simulink model "comm_test"  (R2021a)
settings: Solver=FixedStepAuto  StartTime=0.0  StopTime=inf  RelTol=1e-3
model workspace (MAT data in the model file):
  SL_ROS_VariableLengthArrays_MaxSizes.CommonInfo.ArrayTruncateAction = 'EmitWarning'
  SL_ROS_VariableLengthArrays_MaxSizes.MsgTypeMap = containers.Map
  SL_ROS_VariableLengthArrays_MaxSizes.MsgTypeMap.serialization.keys = {'ambf_walker/DesiredJoints', 'sensor_msgs/JointState'}
  SL_ROS_VariableLengthArrays_MaxSizes.MsgTypeMap.serialization.values{1}(1).PropertyName = 'Controller'
  SL_ROS_VariableLengthArrays_MaxSizes.MsgTypeMap.serialization.values{1}(1).DataType = 'uint8'
  SL_ROS_VariableLengthArrays_MaxSizes.MsgTypeMap.serialization.values{1}(1).MaxLength = 128
  SL_ROS_VariableLengthArrays_MaxSizes.MsgTypeMap.serialization.values{1}(2).PropertyName = 'Other'
  SL_ROS_VariableLengthArrays_MaxSizes.MsgTypeMap.serialization.values{1}(2).DataType = 'double'
  SL_ROS_VariableLengthArrays_MaxSizes.MsgTypeMap.serialization.values{1}(2).MaxLength = 7
  SL_ROS_VariableLengthArrays_MaxSizes.MsgTypeMap.serialization.values{1}(3).PropertyName = 'Q'
  SL_ROS_VariableLengthArrays_MaxSizes.MsgTypeMap.serialization.values{1}(3).DataType = 'double'
  SL_ROS_VariableLengthArrays_MaxSizes.MsgTypeMap.serialization.values{1}(3).MaxLength = 7
  SL_ROS_VariableLengthArrays_MaxSizes.MsgTypeMap.serialization.values{1}(4).PropertyName = 'Qd'
  SL_ROS_VariableLengthArrays_MaxSizes.MsgTypeMap.serialization.values{1}(4).DataType = 'double'
  SL_ROS_VariableLengthArrays_MaxSizes.MsgTypeMap.serialization.values{1}(4).MaxLength = 7
  SL_ROS_VariableLengthArrays_MaxSizes.MsgTypeMap.serialization.values{1}(5).PropertyName = 'Qdd'
  SL_ROS_VariableLengthArrays_MaxSizes.MsgTypeMap.serialization.values{1}(5).DataType = 'double'
  SL_ROS_VariableLengthArrays_MaxSizes.MsgTypeMap.serialization.values{1}(5).MaxLength = 7
  SL_ROS_VariableLengthArrays_MaxSizes.MsgTypeMap.serialization.values{2}(1).PropertyName = 'Effort'
  SL_ROS_VariableLengthArrays_MaxSizes.MsgTypeMap.serialization.values{2}(1).DataType = 'double'
  SL_ROS_VariableLengthArrays_MaxSizes.MsgTypeMap.serialization.values{2}(1).MaxLength = 7
  SL_ROS_VariableLengthArrays_MaxSizes.MsgTypeMap.serialization.values{2}(2).PropertyName = 'Name'
  SL_ROS_VariableLengthArrays_MaxSizes.MsgTypeMap.serialization.values{2}(2).DataType = 'std_msgs/String'
  SL_ROS_VariableLengthArrays_MaxSizes.MsgTypeMap.serialization.values{2}(2).MaxLength = 7
  SL_ROS_VariableLengthArrays_MaxSizes.MsgTypeMap.serialization.values{2}(3).PropertyName = 'Position'
  SL_ROS_VariableLengthArrays_MaxSizes.MsgTypeMap.serialization.values{2}(3).DataType = 'double'
  SL_ROS_VariableLengthArrays_MaxSizes.MsgTypeMap.serialization.values{2}(3).MaxLength = 7
  SL_ROS_VariableLengthArrays_MaxSizes.MsgTypeMap.serialization.values{2}(4).PropertyName = 'Velocity'
  SL_ROS_VariableLengthArrays_MaxSizes.MsgTypeMap.serialization.values{2}(4).DataType = 'double'
  SL_ROS_VariableLengthArrays_MaxSizes.MsgTypeMap.serialization.values{2}(4).MaxLength = 7
  SL_ROS_VariableLengthArrays_MaxSizes.MsgTypeMap.serialization.uniformity = 0
  SL_ROS_VariableLengthArrays_MaxSizes.MsgTypeMap.serialization.keyType = 'char'
  SL_ROS_VariableLengthArrays_MaxSizes.MsgTypeMap.serialization.valueType = 'any'
values from neighbouring files (symbols this model uses):
  Kd = eye(7)*10    [PD_controller_setup.m]    (also in sliding_controller_init.m = 50*eye(7))
  Kp = eye(7)*10    [PD_controller_setup.m]
libraries: robotlib x12
settings Model: Creator=nathanielgoldfarb  LastModifiedBy=nathanielgoldfarb
settings OptimizationCC: EnhancedBackFolding=on  PassReuseOutputArgsAs=Individual arguments  ZeroExternalMemoryAtStartup=off  ZeroInternalMemoryAtStartup=off  MaxStackSize=64  OptimizeBlockOrder=speed  DifferentSizesBufferReuse=on  OptimizationCustomize=off  EfficientTunableParamExpr=on
settings DebuggingCC: ParameterTunabilityLossMsg=error
settings HardwareCC: ProdBitPerPointer=32  ProdBitPerSizeT=32  ProdBitPerPtrDiffT=32  ProdLargestAtomicFloat=None  ProdIntDivRoundTo=Undefined  ProdEndianess=Unspecified  ProdWordSize=32  ProdHWDeviceType=Generic->Unspecified (assume 32-bit Generic)  UseEmbeddedCoderFeatures=off
settings SFSimCC: MATLABDynamicMemAlloc=off
settings RTWCC: SystemTargetFile=ert.tlc  HardwareBoard=Robot Operating System (ROS)  TLCOptions="-aInlineSetEventsForThisBaseRateFcn=TLC_FALSE -aSuppressMultiTaskScheduler=TLC_FALSE  -aRateBasedStepFcn=0"  TemplateMakefile=ert_default_tmf  Toolchain=Catkin  TargetLang=C++
settings CodeAppCC: ForceParamTrailComments=on  IgnoreCustomStorageClasses=off  OperatorAnnotations=on  SimulinkDataObjDesc=on  SFDataObjDesc=on  InsertBlockDesc=on
settings ERTTargetCC: SupportNonInlinedSFcns=on

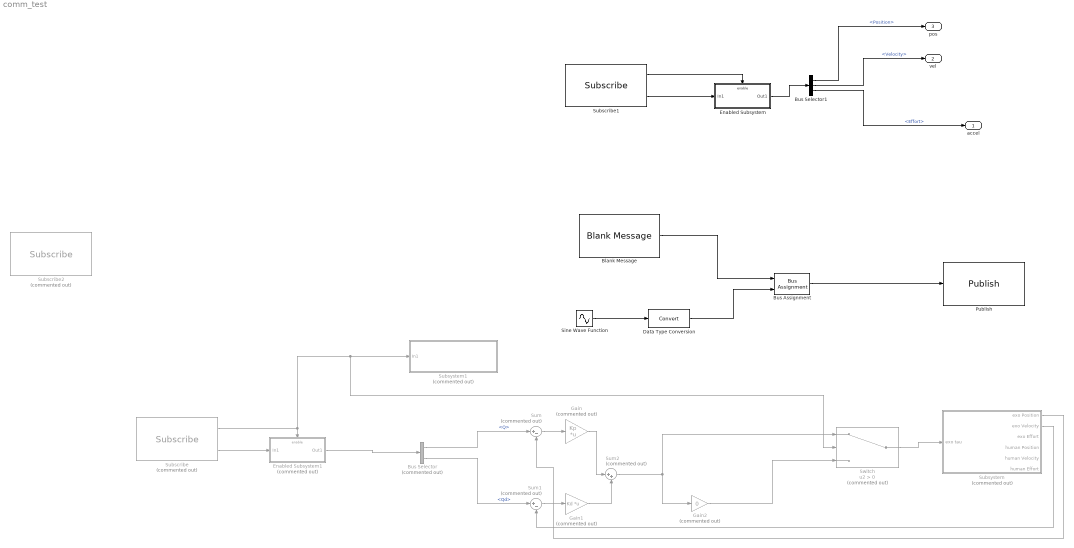
== system comm_test ==
  Blank Message : robotlib/Blank Message  messageClass=Message  entityType=std_msgs/Float32  messageType=std_msgs/Float32  SampleTime=-1  legacyBusStruct=off
  Bus Assignment : BusAssignment  AssignedSignals=Data
  Bus Selector : BusSelector  Commented=on  OutputSignals=Q,Qd
  Bus Selector1 : BusSelector  OutputSignals=Position,Velocity,Effort
  Data Type Conversion : DataTypeConversion
  Enabled Subsystem : Subsystem  TreatAsAtomicUnit=on
  Enabled Subsystem1 : Subsystem  Commented=on  TreatAsAtomicUnit=on
  Gain : Gain  Commented=on  Gain=Kp  Multiplication=Matrix(K*u)
  Gain1 : Gain  Commented=on  Gain=Kd  Multiplication=Matrix(K*u)
  Gain2 : Gain  Commented=on  Gain=0
  Publish : robotlib/Publish  topicSource=Specify your own  topic=/sin_wave  messageType=std_msgs/Float32  legacyBusStruct=off  messageQueueLength=1
  Sine Wave Function : Sin  SampleTime=0
  Subscribe : robotlib/Subscribe  Commented=on  topicSource=Select from ROS network  topic=/exosimulink_set_points  messageType=ambf_walker/DesiredJoints  SampleTime=-1  legacyBusStruct=off  messageQueueLength=1
  Subscribe1 : robotlib/Subscribe  topicSource=Select from ROS network  topic=/exo_jointstate  messageType=sensor_msgs/JointState  SampleTime=-1  legacyBusStruct=off  messageQueueLength=1
  Subscribe2 : robotlib/Subscribe  Commented=on  topicSource=Select from ROS network  topic=/exo_jointstate  messageType=sensor_msgs/JointState  SampleTime=-1  legacyBusStruct=off  messageQueueLength=1
  Subsystem : Subsystem  Commented=on
  Subsystem1 : Subsystem  Commented=on
  Sum : Sum  Commented=on  Inputs=|+-
  Sum1 : Sum  Commented=on  Inputs=|+-
  Sum2 : Sum  Commented=on  Inputs=|++
  Switch : Switch  Commented=on  Criteria=u2 > Threshold
  accel : Outport
  vel : Outport  Port=2
  pos : Outport  Port=3
  wires:
  Subscribe/2 -> Enabled Subsystem1/1(In1)
  Subscribe/1 -> Switch/2, Subsystem1/1(In1), Enabled Subsystem1/Enable
  Sum/1 -> Gain/1
  Sum1/1 -> Gain1/1
  Subsystem/1(exo Position) -> Sum/2
  Subsystem/2(exo Velocity) -> Sum1/2
  Gain/1 -> Sum2/1
  Gain1/1 -> Sum2/2
  Bus Selector/1 -> Sum/1  "<Q>"
  Bus Selector/2 -> Sum1/1  "<Qd>"
  Bus Assignment/1 -> Publish/1
  Blank Message/1 -> Bus Assignment/1
  Sine Wave Function/1 -> Data Type Conversion/1
  Data Type Conversion/1 -> Bus Assignment/2
  Enabled Subsystem1/1(Out1) -> Bus Selector/1
  Sum2/1 -> Switch/1, Gain2/1
  Switch/1 -> Subsystem/1(exo tau)
  Gain2/1 -> Switch/3
  Bus Selector1/1 -> pos/1  "<Position>"
  Subscribe1/1 -> Enabled Subsystem/Enable
  Enabled Subsystem/1(Out1) -> Bus Selector1/1
  Subscribe1/2 -> Enabled Subsystem/1(In1)
  Bus Selector1/3 -> accel/1  "<Effort>"
  Bus Selector1/2 -> vel/1  "<Velocity>"

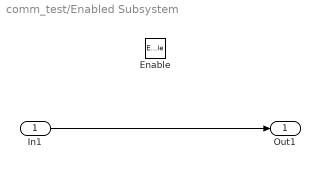
== system comm_test/Enabled Subsystem ==
  In1 : Inport
  Enable : EnablePort
  Out1 : Outport
  wires:
  In1/1 -> Out1/1

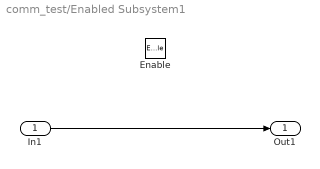
== system comm_test/Enabled Subsystem1 ==
  In1 : Inport
  Enable : EnablePort
  Out1 : Outport
  wires:
  In1/1 -> Out1/1

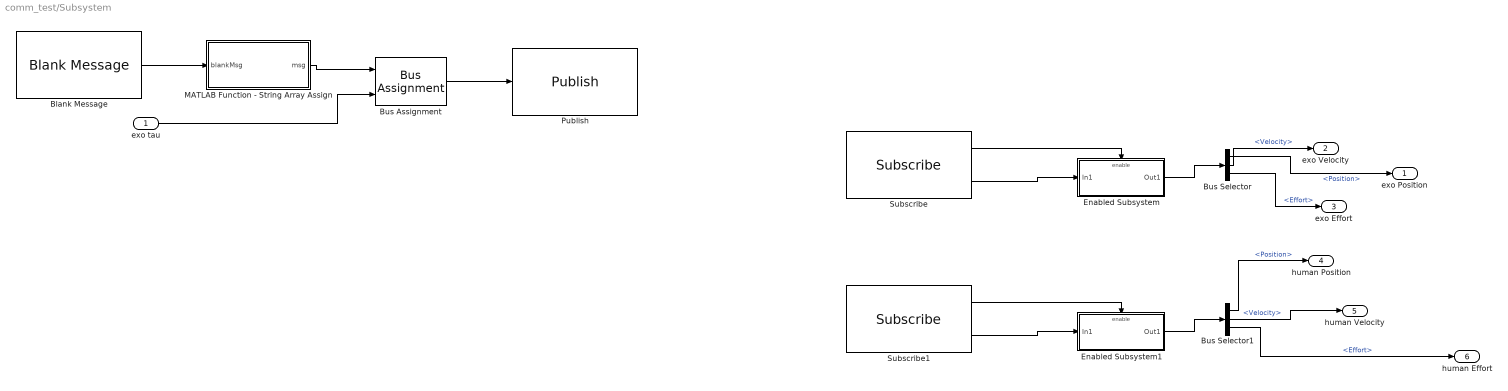
== system comm_test/Subsystem ==
  exo tau : Inport
  Blank Message : robotlib/Blank Message  messageClass=Message  entityType=sensor_msgs/JointState  messageType=sensor_msgs/JointState  SampleTime=inf  legacyBusStruct=off
  Bus Assignment : BusAssignment  AssignedSignals=Effort
  Bus Selector : BusSelector  OutputSignals=Position,Velocity,Effort
  Bus Selector1 : BusSelector  OutputSignals=Position,Velocity,Effort
  Enabled Subsystem : Subsystem  TreatAsAtomicUnit=on
  Enabled Subsystem1 : Subsystem  TreatAsAtomicUnit=on
  MATLAB Function - String Array Assign : MATLAB Function  TreatAsAtomicUnit=on
  Publish : robotlib/Publish  topicSource=Specify your own  topic=/simulink_jointstate  messageType=sensor_msgs/JointState  legacyBusStruct=off  messageQueueLength=1
  Subscribe : robotlib/Subscribe  topicSource=Select from ROS network  topic=/exo_jointstate  messageType=sensor_msgs/JointState  SampleTime=-1  legacyBusStruct=off  messageQueueLength=1
  Subscribe1 : robotlib/Subscribe  topicSource=Select from ROS network  topic=/human_jointstate  messageType=sensor_msgs/JointState  SampleTime=-1  legacyBusStruct=off  messageQueueLength=1
  exo Position : Outport
  exo Velocity : Outport  Port=2
  exo Effort : Outport  Port=3
  human Position : Outport  Port=4
  human Velocity : Outport  Port=5
  human Effort : Outport  Port=6
  wires:
  Enabled Subsystem1/1(Out1) -> Bus Selector1/1
  Subscribe1/2 -> Enabled Subsystem1/1(In1)
  Blank Message/1 -> MATLAB Function - String Array Assign/1(blankMsg)
  Subscribe/1 -> Enabled Subsystem/Enable
  Bus Selector1/1 -> human Position/1  "<Position>"
  Bus Selector/1 -> exo Position/1  "<Position>"
  Subscribe/2 -> Enabled Subsystem/1(In1)
  Bus Selector/2 -> exo Velocity/1  "<Velocity>"
  Bus Selector1/2 -> human Velocity/1  "<Velocity>"
  Enabled Subsystem/1(Out1) -> Bus Selector/1
  Bus Selector/3 -> exo Effort/1  "<Effort>"
  Bus Selector1/3 -> human Effort/1  "<Effort>"
  Subscribe1/1 -> Enabled Subsystem1/Enable
  exo tau/1 -> Bus Assignment/2
  Bus Assignment/1 -> Publish/1
  MATLAB Function - String Array Assign/1(msg) -> Bus Assignment/1

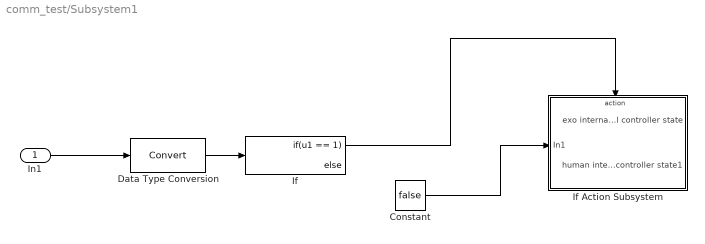
== system comm_test/Subsystem1 ==
  In1 : Inport
  Constant : Constant  Value=false
  Data Type Conversion : DataTypeConversion
  If : If  IfExpression=u1 == 1
  If Action Subsystem : Subsystem  TreatAsAtomicUnit=on
  wires:
  In1/1 -> Data Type Conversion/1
  If/1 -> If Action Subsystem/Action
  Data Type Conversion/1 -> If/1
  Constant/1 -> If Action Subsystem/1(In1)

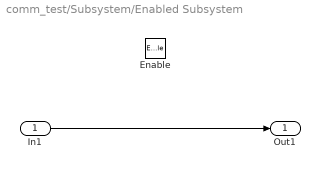
== system comm_test/Subsystem/Enabled Subsystem ==
  In1 : Inport
  Enable : EnablePort
  Out1 : Outport
  wires:
  In1/1 -> Out1/1

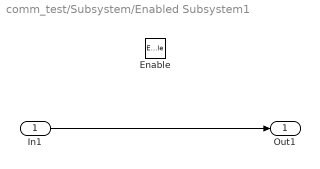
== system comm_test/Subsystem/Enabled Subsystem1 ==
  In1 : Inport
  Enable : EnablePort
  Out1 : Outport
  wires:
  In1/1 -> Out1/1

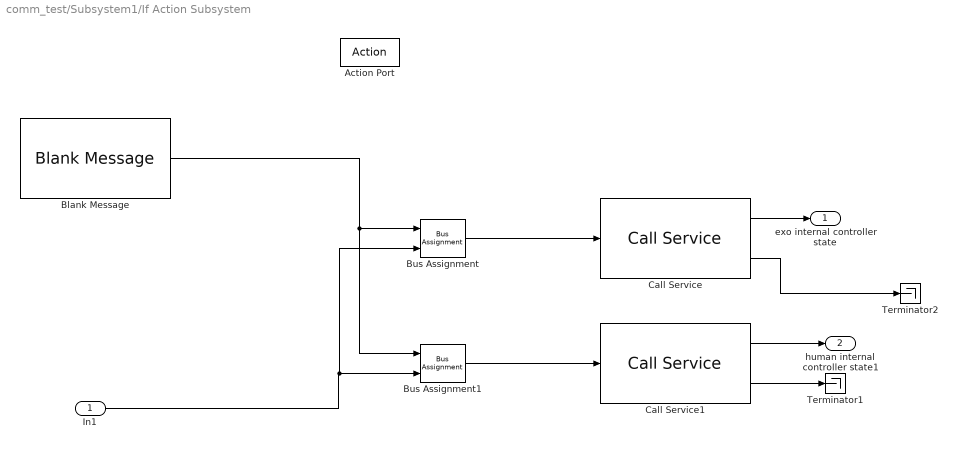
== system comm_test/Subsystem1/If Action Subsystem ==
  In1 : Inport
  Action Port : ActionPort  ActionPortLabel=if(u1 == 1)
  Blank Message : robotlib/Blank Message  messageClass=Service Request  entityType=std_srvs/SetBool  messageType=std_srvs/SetBoolRequest  SampleTime=inf  legacyBusStruct=off
  Bus Assignment : BusAssignment  AssignedSignals=Data
  Bus Assignment1 : BusAssignment  AssignedSignals=Data
  Call Service : robotlib/Call Service  topicSource=Select from ROS network  service=/exo_controller_onoff  serviceType=std_srvs/SetBool  connectionTimeout=5  keepPersistent=on  ShowErrorCodeOutput=on  legacyBusStruct=off
      settings: SourceProductBaseCode=RR
  Call Service1 : robotlib/Call Service  topicSource=Select from ROS network  service=/human_controller_onoff  serviceType=std_srvs/SetBool  connectionTimeout=5  keepPersistent=on  ShowErrorCodeOutput=on  legacyBusStruct=off
      settings: SourceProductBaseCode=RR
  Terminator1 : Terminator
  Terminator2 : Terminator
  exo internal controller state : Outport
  human internal controller state1 : Outport  Port=2
  wires:
  In1/1 -> Bus Assignment/2, Bus Assignment1/2
  Bus Assignment1/1 -> Call Service1/1
  Call Service/1 -> exo internal controller state/1
  Bus Assignment/1 -> Call Service/1
  Call Service/2 -> Terminator2/1
  Blank Message/1 -> Bus Assignment1/1, Bus Assignment/1
  Call Service1/1 -> human internal controller state1/1
  Call Service1/2 -> Terminator1/1

== matlab function comm_test/Subsystem/MATLAB Function - String Array Assign ==
  data: blankMsg input; msg output Bus: SL_Bus_comm_test_sensor_msgs_JointState
function msg = stringArrayAssign(blankMsg)
% stringArrayAssign - Assign a string array in a ROS message
%
%  blankMsg (input): A bus for a 'sensor_msgs/JointState' message. This is 
%      used to initialize the output.
%  msg (output): A bus for a 'sensor_msgs/JointState' message message, with 
%      Name field set to a string array.
%
%   Copyright 2015 The MathWorks, Inc.

%#codegen

% Note: The datatype of 'msg' has been explicitly set to the appropriate 
% Simulink bus type ("SL_Bus_robotROSMessageUsageExample_sensor_msgs_JointState"). 
%
% If the model name is changed, the datatype needs to be changed as well:
%   1) Click "Edit Data" in the Editor toolstrip to open "Ports and Data Manager"
%   2) Select "msg". From the "Type" dropdown, select "--- Refresh data types ---"
%   3) Set datatype to "Bus: SL_Bus_<modelname>_sensor_msgs_JointState"

strArrayToAssign = {'LeftHip', 'LeftKnee', 'LeftAnkle', 'RightHip', 'RightKnee', 'RightAnkle', 'Crutches'};
msg = blankMsg;

% Set the number of strings in the string array.
% msg (sensor_msgs/JointState) includes the following fields
%           Name : array of std_msgs/String (string array)
%   Name_SL_Info : struct with fields CurrentLength, ReceivedLength
numStringsInArray = length(strArrayToAssign);
msg.Name_SL_Info.CurrentLength = uint32(numStringsInArray);
msg.Effort_SL_Info.CurrentLength = uint32(numStringsInArray);

% Set the individual strings in the array
for idx=1:numStringsInArray
    str = strArrayToAssign{idx};
    strLength = length(str);
    msg.Name(idx).Data(1:strLength) = uint8(str);
    msg.Name(idx).Data_SL_Info.CurrentLength = uint32(strLength);
end
